simulink library "SepehrMILLib"  (R2022a)
settings: Solver=VariableStepAuto  StartTime=0.0  StopTime=10.0  RelTol=1e-3
values from neighbouring files (symbols this model uses):
  visSampleTime = 0.1    [SPARCS_MIL_init.m]
undefined symbols (not defined in the file or in its folder): attitude, epoch, IAU, km, m, s, satellite, simulator, WMM2020
libraries: sharedtransform x14, aerolibconvert2 x11, aerolibutil x7, simulink_extras x5, vrlib x4, aerolibtransform2 x3, sharedutil x3, aerolibgravity2 x2, aerolibcelestial x2, aerolibobsolete x1, aerolibattitudesys x1, simulink x1
(part 2 of 2)

== system SepehrMILLib/Reference Frames Transformations Manager/Quaternion Conditioner11 ==
  Q : Inport  PortDimensions=[4,1]
  Interpreted MATLAB Function : MATLABFcn  MATLABFcn=[u(1),0,0,0;0,u(2),0,0;0,0,u(3),0;0,0,0,u(4)]
  Interpreted MATLAB Function1 : MATLABFcn  MATLABFcn=[u(1),0,0,0;0,u(2),0,0;0,0,u(3),0;0,0,0,u(4)]
  Interpreted MATLAB Function2 : MATLABFcn  MATLABFcn=(u(1)+u(6)+u(11)+u(16))+1.9
  Product : Product
  Product1 : Product
  Sign : Signum
  Sign1 : Signum
  Unit Delay : UnitDelay  InitialCondition=[1;0;0;0]  SampleTime=-1  HasFrameUpgradeWarning=on
  Qc : Outport  PortDimensions=[4,1]
  wires:
  Interpreted MATLAB Function2/1 -> Sign1/1
  Product1/1 -> Unit Delay/1, Qc/1
  Interpreted MATLAB Function/1 -> Product/1
  Product/1 -> Sign/1
  Sign/1 -> Interpreted MATLAB Function2/1
  Interpreted MATLAB Function1/1 -> Product/2
  Sign1/1 -> Product1/2
  Unit Delay/1 -> Interpreted MATLAB Function1/1
  Q/1 -> Product1/1, Interpreted MATLAB Function/1

== system SepehrMILLib/Reference Frames Transformations Manager/Quaternion Conditioner6 ==
  Q : Inport  PortDimensions=[4,1]
  Interpreted MATLAB Function : MATLABFcn  MATLABFcn=[u(1),0,0,0;0,u(2),0,0;0,0,u(3),0;0,0,0,u(4)]
  Interpreted MATLAB Function1 : MATLABFcn  MATLABFcn=[u(1),0,0,0;0,u(2),0,0;0,0,u(3),0;0,0,0,u(4)]
  Interpreted MATLAB Function2 : MATLABFcn  MATLABFcn=(u(1)+u(6)+u(11)+u(16))+1.9
  Product : Product
  Product1 : Product
  Sign : Signum
  Sign1 : Signum
  Unit Delay : UnitDelay  InitialCondition=[1;0;0;0]  SampleTime=-1  HasFrameUpgradeWarning=on
  Qc : Outport  PortDimensions=[4,1]
  wires:
  Q/1 -> Interpreted MATLAB Function/1, Product1/1
  Unit Delay/1 -> Interpreted MATLAB Function1/1
  Sign1/1 -> Product1/2
  Interpreted MATLAB Function1/1 -> Product/2
  Sign/1 -> Interpreted MATLAB Function2/1
  Product/1 -> Sign/1
  Interpreted MATLAB Function/1 -> Product/1
  Product1/1 -> Qc/1, Unit Delay/1
  Interpreted MATLAB Function2/1 -> Sign1/1

== system SepehrMILLib/Reference Frames Transformations Manager/Quaternion Conditioner7 ==
  Q : Inport  PortDimensions=[4,1]
  Interpreted MATLAB Function : MATLABFcn  MATLABFcn=[u(1),0,0,0;0,u(2),0,0;0,0,u(3),0;0,0,0,u(4)]
  Interpreted MATLAB Function1 : MATLABFcn  MATLABFcn=[u(1),0,0,0;0,u(2),0,0;0,0,u(3),0;0,0,0,u(4)]
  Interpreted MATLAB Function2 : MATLABFcn  MATLABFcn=(u(1)+u(6)+u(11)+u(16))+1.9
  Product : Product
  Product1 : Product
  Sign : Signum
  Sign1 : Signum
  Unit Delay : UnitDelay  InitialCondition=[1;0;0;0]  SampleTime=-1  HasFrameUpgradeWarning=on
  Qc : Outport  PortDimensions=[4,1]
  wires:
  Interpreted MATLAB Function2/1 -> Sign1/1
  Product1/1 -> Unit Delay/1, Qc/1
  Interpreted MATLAB Function/1 -> Product/1
  Product/1 -> Sign/1
  Sign/1 -> Interpreted MATLAB Function2/1
  Interpreted MATLAB Function1/1 -> Product/2
  Sign1/1 -> Product1/2
  Unit Delay/1 -> Interpreted MATLAB Function1/1
  Q/1 -> Product1/1, Interpreted MATLAB Function/1

== system SepehrMILLib/Reference Frames Transformations Manager/Quaternion Conditioner8 ==
  Q : Inport  PortDimensions=[4,1]
  Interpreted MATLAB Function : MATLABFcn  MATLABFcn=[u(1),0,0,0;0,u(2),0,0;0,0,u(3),0;0,0,0,u(4)]
  Interpreted MATLAB Function1 : MATLABFcn  MATLABFcn=[u(1),0,0,0;0,u(2),0,0;0,0,u(3),0;0,0,0,u(4)]
  Interpreted MATLAB Function2 : MATLABFcn  MATLABFcn=(u(1)+u(6)+u(11)+u(16))+1.9
  Product : Product
  Product1 : Product
  Sign : Signum
  Sign1 : Signum
  Unit Delay : UnitDelay  InitialCondition=[1;0;0;0]  SampleTime=-1  HasFrameUpgradeWarning=on
  Qc : Outport  PortDimensions=[4,1]
  wires:
  Q/1 -> Interpreted MATLAB Function/1, Product1/1
  Unit Delay/1 -> Interpreted MATLAB Function1/1
  Sign1/1 -> Product1/2
  Interpreted MATLAB Function1/1 -> Product/2
  Sign/1 -> Interpreted MATLAB Function2/1
  Product/1 -> Sign/1
  Interpreted MATLAB Function/1 -> Product/1
  Product1/1 -> Qc/1, Unit Delay/1
  Interpreted MATLAB Function2/1 -> Sign1/1

== system SepehrMILLib/Reference Frames Transformations Manager/Quaternion Conditioner9 ==
  Q : Inport  PortDimensions=[4,1]
  Interpreted MATLAB Function : MATLABFcn  MATLABFcn=[u(1),0,0,0;0,u(2),0,0;0,0,u(3),0;0,0,0,u(4)]
  Interpreted MATLAB Function1 : MATLABFcn  MATLABFcn=[u(1),0,0,0;0,u(2),0,0;0,0,u(3),0;0,0,0,u(4)]
  Interpreted MATLAB Function2 : MATLABFcn  MATLABFcn=(u(1)+u(6)+u(11)+u(16))+1.9
  Product : Product
  Product1 : Product
  Sign : Signum
  Sign1 : Signum
  Unit Delay : UnitDelay  InitialCondition=[1;0;0;0]  SampleTime=-1  HasFrameUpgradeWarning=on
  Qc : Outport  PortDimensions=[4,1]
  wires:
  Interpreted MATLAB Function2/1 -> Sign1/1
  Product1/1 -> Unit Delay/1, Qc/1
  Interpreted MATLAB Function/1 -> Product/1
  Product/1 -> Sign/1
  Sign/1 -> Interpreted MATLAB Function2/1
  Interpreted MATLAB Function1/1 -> Product/2
  Sign1/1 -> Product1/2
  Unit Delay/1 -> Interpreted MATLAB Function1/1
  Q/1 -> Product1/1, Interpreted MATLAB Function/1

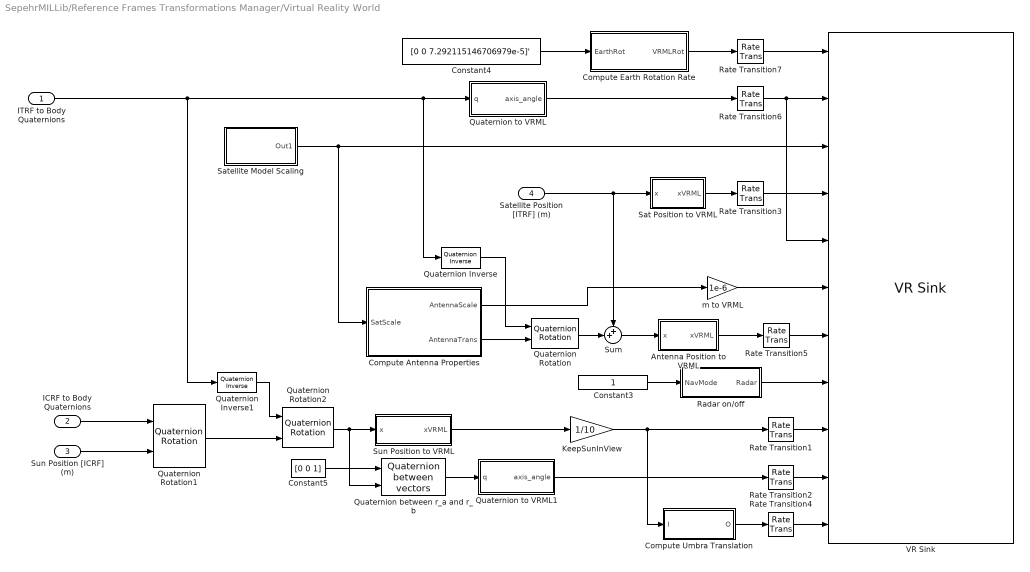
== system SepehrMILLib/Reference Frames Transformations Manager/Virtual Reality World ==
  ITRF to Body Quaternions : Inport
  ICRF to Body Quaternions : Inport  Port=2
  Sun Position [ICRF] (m) : Inport  Port=3
  Satellite Position [ITRF] (m) : Inport  Port=4
  Antenna Position to VRML : Subsystem
  Compute Antenna Properties : Subsystem
  Compute Earth Rotation Rate : Subsystem
  Compute Umbra Translation : Subsystem
  Constant3 : Constant
  Constant4 : Constant  Value=[0 0 7.292115146706979e-5]'
  Constant5 : Constant  Value=[0 0 1]
  KeepSunInView : Gain  Gain=1/10
  Quaternion Inverse : aerolibutil/Quaternion Inverse
  Quaternion Inverse1 : aerolibutil/Quaternion Inverse
  Quaternion Rotation : aerolibutil/Quaternion Rotation
  Quaternion Rotation1 : aerolibutil/Quaternion Rotation
  Quaternion Rotation2 : aerolibutil/Quaternion Rotation
  Quaternion between r_a and r_b : aerolibattitudesys/Quaternion between vectors
      settings: SourceProductBaseCode=AE
  Quaternion to VRML : Subsystem
  Quaternion to VRML1 : Subsystem
  Radar on/off : Subsystem
  Rate Transition{1..7} (7 alike) : RateTransition
  Sat Position to VRML : Subsystem
  Satellite Model Scaling : Subsystem
  Sum : Sum  Inputs=++|
  Sun Position to VRML : Subsystem
  VR Sink : vrlib/VR Sink  InstantiateOnLoad=on  SampleTime=visSampleTime  ViewEnable=on  RemoteChange=off  RemoteView=off  FieldsWritten=Earth.rotation.4.1.1.double#Satellite.rotation.4.1.1.double#Satellite.scale.3.1.1.double#Satellite.translation.3.1.1.double#AntennaCone.rotation.4.1.1.double#AntennaCone.scale.3.1.1.double#AntennaCone.translation.3.1.1.double#AntennaMaterial.transparency.1.1.1.double#Sun.translation.3.1.1.double#Umbra.rotation.4.1.1.double#Umbra.translation.3.1.1.double  WorldFileName=cubesatAnim.wrl  WorldDescription=CubeSat Orbit Animation  AutoView=on  VideoDimensions=[]  AllowVariableSize=off
  m to VRML : Gain  Gain=1e-6
  wires:
  ITRF to Body Quaternions/1 -> Quaternion to VRML/1(q), Quaternion Inverse/1, Quaternion Inverse1/1
  Constant3/1 -> Radar on/off/1(NavMode)
  Satellite Position [ITRF] (m)/1 -> Sat Position to VRML/1(x), Sum/1
  Quaternion Inverse/1 -> Quaternion Rotation/1
  Sum/1 -> Antenna Position to VRML/1(x)
  Quaternion Rotation/1 -> Sum/2
  Quaternion Rotation2/1 -> Sun Position to VRML/1(x), Quaternion between r_a and r_b/2
  Quaternion Rotation1/1 -> Quaternion Rotation2/2
  Quaternion Inverse1/1 -> Quaternion Rotation2/1
  Sun Position to VRML/1(xVRML) -> KeepSunInView/1
  Quaternion between r_a and r_b/1 -> Quaternion to VRML1/1(q)
  Constant5/1 -> Quaternion between r_a and r_b/1
  m to VRML/1 -> VR Sink/6
  Antenna Position to VRML/1(xVRML) -> Rate Transition5/1
  Compute Earth Rotation Rate/1(VRMLRot) -> Rate Transition7/1
  Sat Position to VRML/1(xVRML) -> Rate Transition3/1
  Radar on/off/1(Radar) -> VR Sink/8
  Quaternion to VRML1/1(axis_angle) -> Rate Transition2/1
  KeepSunInView/1 -> Compute Umbra Translation/1(I), Rate Transition1/1
  Compute Umbra Translation/1(O) -> Rate Transition4/1
  Satellite Model Scaling/1(Out1) -> VR Sink/3, Compute Antenna Properties/1(SatScale)
  Compute Antenna Properties/1(AntennaScale) -> m to VRML/1
  Compute Antenna Properties/2(AntennaTrans) -> Quaternion Rotation/2
  ICRF to Body Quaternions/1 -> Quaternion Rotation1/1
  Sun Position [ICRF] (m)/1 -> Quaternion Rotation1/2
  Rate Transition4/1 -> VR Sink/11
  Rate Transition1/1 -> VR Sink/9
  Rate Transition2/1 -> VR Sink/10
  Constant4/1 -> Compute Earth Rotation Rate/1(EarthRot)
  Rate Transition7/1 -> VR Sink/1
  Rate Transition3/1 -> VR Sink/4
  Rate Transition5/1 -> VR Sink/7
  Quaternion to VRML/1(axis_angle) -> Rate Transition6/1
  Rate Transition6/1 -> VR Sink/5, VR Sink/2

== system SepehrMILLib/Reference Frames Transformations Manager/Virtual Reality World/Antenna Position to VRML ==
  x : Inport
  ECEF to VRML : Subsystem
  Length Conversion : aerolibconvert2/Length Conversion  IU=m  OU=km
  km to VRML units : Gain  Gain=1/1000
  xVRML : Outport  VectorParamsAs1DForOutWhenUnconnected=off
  wires:
  Length Conversion/1 -> km to VRML units/1
  km to VRML units/1 -> ECEF to VRML/1(M)
  x/1 -> Length Conversion/1
  ECEF to VRML/1(VR) -> xVRML/1

== system SepehrMILLib/Reference Frames Transformations Manager/Virtual Reality World/Compute Antenna Properties ==
  SatScale : Inport
  Constant1 : Constant  Value=25
  Constant2 : Constant  Value=1e6
  Constant4 : Constant  Value=0
  Gain1 : Gain  Gain=.5
  Gain2 : Gain  Gain=pi/180
  Mux1 : Mux  Inputs=3
  Mux2 : Mux  Inputs=3
  Product : Product
  Selector : Selector  InputPortWidth=3  IndexOptions=Index vector (dialog)  Indices=1  OutputSizes=1
  Sum1 : Sum  Inputs=++|
  Trigonometric Function : Trigonometry  Operator=tan
  gain : Gain  Gain=.25*1e6
  AntennaScale : Outport  VectorParamsAs1DForOutWhenUnconnected=off
  AntennaTrans : Outport  Port=2  VectorParamsAs1DForOutWhenUnconnected=off
  wires:
  Gain2/1 -> Trigonometric Function/1
  Constant4/1 -> Mux2/1, Mux2/2
  Sum1/1 -> Mux2/3
  Constant2/1 -> Gain1/1, Mux1/2, Product/2
  gain/1 -> Sum1/1
  Constant1/1 -> Gain2/1
  Product/1 -> Mux1/3, Mux1/1
  Gain1/1 -> Sum1/2
  Trigonometric Function/1 -> Product/1
  Mux2/1 -> AntennaTrans/1
  Mux1/1 -> AntennaScale/1
  SatScale/1 -> Selector/1
  Selector/1 -> gain/1

== system SepehrMILLib/Reference Frames Transformations Manager/Virtual Reality World/Compute Earth Rotation Rate ==
  EarthRot : Inport
  Euler Angles to Quaternions : aerolibobsolete/Euler Angles to Quaternions
      settings: SourceProductBaseCode=AE
  Quaternion to VRML : Subsystem
  Sum : Sum  Inputs=|++
  Unit Delay : UnitDelay  SampleTime=-1  HasFrameUpgradeWarning=on
  VRMLRot : Outport  VectorParamsAs1DForOutWhenUnconnected=off
  wires:
  EarthRot/1 -> Sum/1
  Unit Delay/1 -> Sum/2
  Sum/1 -> Unit Delay/1, Euler Angles to Quaternions/1
  Euler Angles to Quaternions/1 -> Quaternion to VRML/1(q)
  Quaternion to VRML/1(AxisAngle) -> VRMLRot/1

== system SepehrMILLib/Reference Frames Transformations Manager/Virtual Reality World/Compute Umbra Translation ==
  I : Inport
  Add : Sum
  ConeHalfLength : Gain  Gain=692
  InvertSunPosECEF : Gain  Gain=-1
  unitVec : Subsystem
  O : Outport  VectorParamsAs1DForOutWhenUnconnected=off
  wires:
  ConeHalfLength/1 -> Add/2
  I/1 -> InvertSunPosECEF/1
  Add/1 -> O/1
  InvertSunPosECEF/1 -> unitVec/1(I), Add/1
  unitVec/1(O) -> ConeHalfLength/1

== system SepehrMILLib/Reference Frames Transformations Manager/Virtual Reality World/Quaternion to VRML ==
  q : Inport
  Demux : Demux
  Flip 180 deg : Constant  Value=[0 0 1 0]
  Gain : Gain  Gain=2
  Mux : Mux
  Quaternion Multiplication : aerolibutil/Quaternion Multiplication
  Selector : Selector  InputPortWidth=4  IndexOptions=Index vector (dialog)  Indices=[3 4 2 1]  OutputSizes=1
  Trigonometric Function : Trigonometry  Operator=acos
  axis_angle : Outport  VectorParamsAs1DForOutWhenUnconnected=off
  wires:
  Demux/4 -> Mux/4
  Demux/3 -> Mux/3
  Demux/2 -> Mux/2
  Gain/1 -> Mux/1
  Selector/1 -> axis_angle/1
  q/1 -> Quaternion Multiplication/1
  Mux/1 -> Selector/1
  Trigonometric Function/1 -> Gain/1
  Demux/1 -> Trigonometric Function/1
  Flip 180 deg/1 -> Quaternion Multiplication/2
  Quaternion Multiplication/1 -> Demux/1

== system SepehrMILLib/Reference Frames Transformations Manager/Virtual Reality World/Quaternion to VRML1 ==
  q : Inport
  Demux : Demux
  Flip 180 deg : Constant  Value=[0 0 1 0]
  Gain : Gain  Gain=2
  Mux : Mux
  Quaternion Multiplication : aerolibutil/Quaternion Multiplication
  Selector : Selector  InputPortWidth=4  IndexOptions=Index vector (dialog)  Indices=[3 4 2 1]  OutputSizes=1
  Trigonometric Function : Trigonometry  Operator=acos
  axis_angle : Outport  VectorParamsAs1DForOutWhenUnconnected=off
  wires:
  Demux/4 -> Mux/4
  Demux/3 -> Mux/3
  Demux/2 -> Mux/2
  Gain/1 -> Mux/1
  Selector/1 -> axis_angle/1
  Mux/1 -> Selector/1
  Trigonometric Function/1 -> Gain/1
  Demux/1 -> Trigonometric Function/1
  Flip 180 deg/1 -> Quaternion Multiplication/2
  q/1 -> Quaternion Multiplication/1
  Quaternion Multiplication/1 -> Demux/1

== system SepehrMILLib/Reference Frames Transformations Manager/Virtual Reality World/Radar on//off ==
  NavMode : Inport
  Add : Sum  Inputs=-+
  Compare To Constant : simulink/Logic and Bit Operations/Compare To Constant  relop===  const=1  OutDataTypeStr=boolean  ZeroCross=off
  Constant : Constant
  Data Type Conversion : DataTypeConversion  OutDataTypeStr=double  SaturateOnIntegerOverflow=off  RndMeth=Floor
  Gain : Gain  Gain=0.6
  Radar : Outport  VectorParamsAs1DForOutWhenUnconnected=off
  wires:
  NavMode/1 -> Compare To Constant/1
  Compare To Constant/1 -> Data Type Conversion/1
  Data Type Conversion/1 -> Gain/1
  Gain/1 -> Add/1
  Constant/1 -> Add/2
  Add/1 -> Radar/1

== system SepehrMILLib/Reference Frames Transformations Manager/Virtual Reality World/Sat Position to VRML ==
  x : Inport
  ECEF to VRML : Subsystem
  Length Conversion : aerolibconvert2/Length Conversion  IU=m  OU=km
  km to VRML units : Gain  Gain=1/1000
  xVRML : Outport  VectorParamsAs1DForOutWhenUnconnected=off
  wires:
  ECEF to VRML/1(VR) -> xVRML/1
  x/1 -> Length Conversion/1
  km to VRML units/1 -> ECEF to VRML/1(M)
  Length Conversion/1 -> km to VRML units/1

== system SepehrMILLib/Reference Frames Transformations Manager/Virtual Reality World/Satellite Model Scaling ==
  Constant : Constant  Value=2e5
  Mux : Mux  Inputs=3
  ScaleModelToVRML : Gain  Gain=1/.3e6
  Out1 : Outport  VectorParamsAs1DForOutWhenUnconnected=off
  wires:
  ScaleModelToVRML/1 -> Mux/3, Mux/1, Mux/2
  Constant/1 -> ScaleModelToVRML/1
  Mux/1 -> Out1/1

== system SepehrMILLib/Reference Frames Transformations Manager/Virtual Reality World/Sun Position to VRML ==
  x : Inport
  ECEF to VRML : Subsystem
  Length Conversion : aerolibconvert2/Length Conversion  IU=m  OU=km
  km to VRML units : Gain  Gain=1/1000
  xVRML : Outport  VectorParamsAs1DForOutWhenUnconnected=off
  wires:
  ECEF to VRML/1(VR) -> xVRML/1
  x/1 -> Length Conversion/1
  km to VRML units/1 -> ECEF to VRML/1(M)
  Length Conversion/1 -> km to VRML units/1

== system SepehrMILLib/Reference Frames Transformations Manager/Virtual Reality World/Antenna Position to VRML/ECEF to VRML ==
  M : Inport  PortDimensions=3
  Selector : Selector  InputPortWidth=3  IndexOptions=Index vector (dialog)  Indices=[2 3 1]  OutputSizes=1
  VR : Outport  PortDimensions=3  VectorParamsAs1DForOutWhenUnconnected=off
  wires:
  M/1 -> Selector/1
  Selector/1 -> VR/1

== system SepehrMILLib/Reference Frames Transformations Manager/Virtual Reality World/Compute Earth Rotation Rate/Quaternion to VRML ==
  q : Inport
  Demux : Demux
  Gain : Gain  Gain=2
  Gain3 : Gain  Gain=[-1 1 1 1]
  Mux : Mux
  Selector : Selector  InputPortWidth=4  IndexOptions=Index vector (dialog)  Indices=[2 4 3 1]  OutputSizes=1
  Trigonometric Function : Trigonometry  Operator=acos
  AxisAngle : Outport  VectorParamsAs1DForOutWhenUnconnected=off
  wires:
  Demux/4 -> Mux/4
  Demux/3 -> Mux/3
  Demux/2 -> Mux/2
  Gain/1 -> Mux/1
  Selector/1 -> Gain3/1
  Gain3/1 -> AxisAngle/1
  q/1 -> Demux/1
  Mux/1 -> Selector/1
  Trigonometric Function/1 -> Gain/1
  Demux/1 -> Trigonometric Function/1

== system SepehrMILLib/Reference Frames Transformations Manager/Virtual Reality World/Compute Umbra Translation/unitVec ==
  I : Inport
  Divide : Product  Inputs=*/
  Dot Product : DotProduct  OutDataTypeStr=Inherit: Inherit via internal rule
  Sqrt : Sqrt
  O : Outport  VectorParamsAs1DForOutWhenUnconnected=off
  wires:
  Dot Product/1 -> Sqrt/1
  I/1 -> Divide/1, Dot Product/1, Dot Product/2
  Divide/1 -> O/1
  Sqrt/1 -> Divide/2

== system SepehrMILLib/Reference Frames Transformations Manager/Virtual Reality World/Sat Position to VRML/ECEF to VRML ==
  M : Inport  PortDimensions=3
  Selector : Selector  InputPortWidth=3  IndexOptions=Index vector (dialog)  Indices=[2 3 1]  OutputSizes=1
  VR : Outport  PortDimensions=3  VectorParamsAs1DForOutWhenUnconnected=off
  wires:
  M/1 -> Selector/1
  Selector/1 -> VR/1

== system SepehrMILLib/Reference Frames Transformations Manager/Virtual Reality World/Sun Position to VRML/ECEF to VRML ==
  M : Inport  PortDimensions=3
  Selector : Selector  InputPortWidth=3  IndexOptions=Index vector (dialog)  Indices=[2 3 1]  OutputSizes=1
  VR : Outport  PortDimensions=3  VectorParamsAs1DForOutWhenUnconnected=off
  wires:
  M/1 -> Selector/1
  Selector/1 -> VR/1

== matlab function SepehrMILLib/Reference Frames Transformations Manager/State Vector to Orbital Elements ==
  data: r input; v input; SemiMajorAxis output; Eccentricity output; Inclination output; RightAscension output; ArgumentOfPerigee output; TrueAnomaly output; mu input; TrueLongitude output; ArgumentOfLatitude output; LongitudeOfPeriapsis output; SemilatusRectum output; OrbOmega output
%----------------------- Begin Code Sequence -----------------------------%
% Purpose:                                                                %
% Convert a given set of state vectors in ECI reference frame to orbital  %
% elements.                                                               %
%-------------------------------------------------------------------------%
%                                                                         %
% Inputs:                                                                 %
%--------                                                                  
%r_ECI                  [3 x N]                         Position Vector in
%                                                       ECI coordinate
%                                                       frame of reference
%
%v_ECI                  [3 x N]                         Velocity vector in
%                                                       ECI coordinate
%                                                       frame of reference
%
%mu                     double                          Gravitational Constant
%                                                       Defaults to Earth if
%                                                       not specified
% Outputs:
%---------                                                                %
%a                      [1 x N]                         Semi-Major Axis
%                                                       (m)
%
%eMag                   [1 x N]                         Eccentricity
%                                                       (unitless)
%
%i                      [1 x N]                         inclination
%                                                       (rad)
%
%O                      [1 x N]                         Right Ascention of
%                                                       the ascending node
%                                                       (rad)
%
%o                      [1 x N]                         Argument of perigee
%                                                       (rad)
%
%M                      [1 x N]                         Mean Anomaly
%                                                       (rad)
%
%truLon                 [1 x N]                         True Longitude
%                                                       (rad)
%
%argLat                 [1 x N]                         Argument of Latitude
%                                                       (rad)
%
%lonPer                 [1 x N]                         Longitude of Periapse
%                                                       (rad)
%
%p                      [1 x N]                         Semilatus Rectum
%                                                       (m)
%
%OrbOmega                                               Orbital Frame
%                                                       angular velocity
%                                                       (rad)
% References:
%-------------
%Vallado,D. Fundamentals of Astrodynamics and Applications. 2007.
%
% Function Dependencies:
%------------------
%None
%------------------------------------------------------------------       %
% Programed by Darin Koblick  03-04-2012                                  %
% modified by A.H.Khodabakhsh 10-01-2021                                  %
% Updated to address circular equatorial orbits       12/12/2013          %
%------------------------------------------------------------------       %
function [SemiMajorAxis,Eccentricity,Inclination,RightAscension,ArgumentOfPerigee,TrueAnomaly,...
          TrueLongitude,ArgumentOfLatitude,LongitudeOfPeriapsis,SemilatusRectum,OrbOmega] = ...
          StateVector2KeplerianOrbitalElemets(r,v,mu)
% if ~exist('mu','var');  t = getConst(); mu = t.Earth.Mu; end
%Specific angular momentum
h = cross(r,v);
n = cross(repmat([0;0;1],[1,size(r,2)]),h); nMag = sqrt(sum(n.^2,1));
vMag = sqrt(sum(v.^2,1)); 
rMag = sqrt(sum(r.^2,1)); 
hMag = sqrt(sum(h.^2,1));
e = (1./mu).*(bsxfun(@times,(vMag.^2 - mu./rMag),r) - bsxfun(@times,dot(r,v),v)); 
Eccentricity = sqrt(sum(e.^2,1));
zeta = (vMag.^2)./2 - mu./rMag;
%Special Procedure when we have a parabolic orbit
idx = Eccentricity ~= 1;
SemiMajorAxis = zeros(size(Eccentricity));
SemilatusRectum = zeros(size(Eccentricity));
if any(idx)
    SemiMajorAxis(idx) = -mu./(2.*zeta(idx)); 
    SemilatusRectum(idx) = SemiMajorAxis(idx).*(1-Eccentricity(idx).^2); 
else
    SemiMajorAxis(idx) = Inf; 
    SemilatusRectum(idx) = (hMag(idx).^2)./mu; 
end
%Compute the angles
Inclination             = acos(double(single(   h(3,:)./hMag)                   )); 
RightAscension          = acos(double(single(   n(1,:)./nMag)                   ));
ArgumentOfPerigee       = acos(double(single(   dot(n,e)./(nMag.*Eccentricity)) ));
TrueAnomaly             = acos(double(single(   dot(e,r)./(Eccentricity.*rMag)) ));
LongitudeOfPeriapsis    = acos(double(single(   e(1,:)./Eccentricity)           ));
ArgumentOfLatitude      = acos(double(single(   dot(n,r)./(nMag.*rMag))         ));
TrueLongitude           = acos(double(single(   r(1,:)./rMag)                   ));
%Account for those cases where satellite is in circular orbit
         RightAscension   (  n(1,:) == 0) = 0;
       ArgumentOfPerigee  (dot(n,e) == 0) = 0;
      LongitudeOfPeriapsis(  e(1,:) == 0) = 0;
          TrueAnomaly     (dot(e,r) == 0) = 0;
       ArgumentOfLatitude (dot(n,r) == 0) = 0;
%Apply Quadrant Checks to All Determined Angles
idx = n(2,:) < 0; if any(idx),  RightAscension(idx) = 2*pi - RightAscension(idx);  end;
idx = e(3,:) < 0; if any(idx), ArgumentOfPerigee(idx) = 2*pi - ArgumentOfPerigee(idx); end;
idx = dot(r,v) < 0; if any(idx), TrueAnomaly(idx) = 2*pi - TrueAnomaly(idx); end;
idx = e(2,:) < 0; if any(idx), LongitudeOfPeriapsis(idx) = 2*pi-LongitudeOfPeriapsis(idx);  end;
idx = r(3,:) < 0; if any(idx), ArgumentOfLatitude(idx) = 2*pi - ArgumentOfLatitude(idx); end;
idx = r(2,:) < 0; if any(idx), TrueLongitude(idx) = 2*pi - TrueLongitude(idx); end;

rv = zeros(3,1);
rv(:)=cross(r,v); norm_r = norm(r);
OrbOmega = [0;
            dot(v,cross(r./norm_r,rv./norm(rv)))/norm_r;
            0];

% % convert radians to degrees
% r2d = @(x) x.*(180./pi);
% Inclination          = r2d(Inclination         );
% RightAscension       = r2d(RightAscension      );
% ArgumentOfPerigee    = r2d(ArgumentOfPerigee   );
% TrueAnomaly          = r2d(TrueAnomaly         );
% TrueLongitude        = r2d(TrueLongitude       );
% ArgumentOfLatitude   = r2d(ArgumentOfLatitude  );
% LongitudeOfPeriapsis = r2d(LongitudeOfPeriapsis);
% OrbOmega             = r2d(OrbOmega            );
end
